simulink model "prob5"  (R2020b)
settings: Solver=VariableStepAuto  StartTime=0.0  StopTime=10.0  RelTol=1e-3
undefined symbols (not defined in the file): C, R
settings Model: Creator=Abhinav dixit  LastModifiedBy=Abhinav dixit

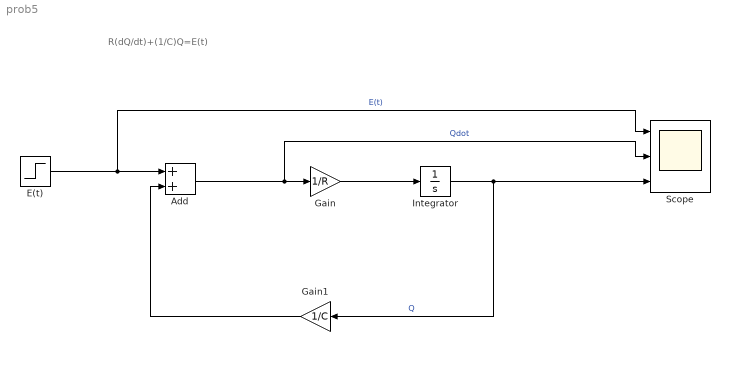
== system prob5 ==
  note: R(dQ/dt)+(1/C)Q=E(t)
  Add : Sum
  E(t) : Step  Before=4  After=5  SampleTime=0
  Gain : Gain  Gain=1/R
  Gain1 : Gain  Gain=1/C
  Integrator : Integrator
  Scope : Scope  NumInputPorts=3
  wires:
  Add/1 -> Scope/2, Gain/1  "Qdot"
  Gain/1 -> Integrator/1
  E(t)/1 -> Scope/1, Add/1  "E(t)"
  Gain1/1 -> Add/2
  Integrator/1 -> Gain1/1, Scope/3  "Q"
